simulink model "for_analysis"  (R2020a)
settings: Solver=VariableStepAuto  StartTime=0.0  StopTime=10.0  RelTol=1e-3
libraries: cstblocks x2
settings Model: Creator=Jason  LastModifiedBy=Jason

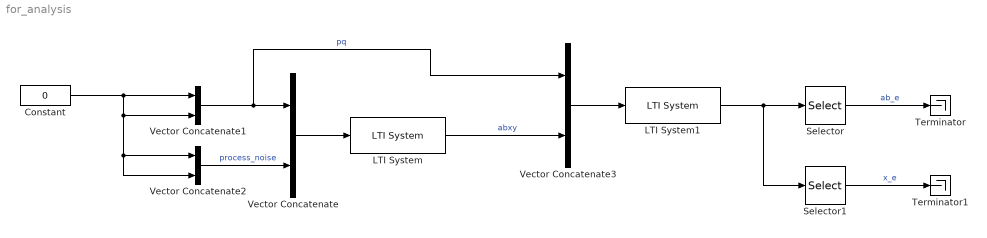
== system for_analysis ==
  Constant : Constant  Value=0
  LTI System : cstblocks/LTI System  sys=sys  IC=[]
  LTI System1 : cstblocks/LTI System  sys=kalmf  IC=[]
  Selector : Selector  InputPortWidth=4  IndexOptions=Index vector (dialog)  Indices=[1 2]  OutputSizes=1
  Selector1 : Selector  InputPortWidth=4  IndexOptions=Index vector (dialog)  Indices=[3 4]  OutputSizes=1
  Terminator : Terminator
  Terminator1 : Terminator
  Vector Concatenate{,1..3} (4 alike) : Concatenate
  wires:
  Vector Concatenate/1 -> LTI System/1
  Vector Concatenate1/1 -> Vector Concatenate3/1, Vector Concatenate/1  "pq"
  Vector Concatenate2/1 -> Vector Concatenate/2  "process_noise"
  Vector Concatenate3/1 -> LTI System1/1
  LTI System/1 -> Vector Concatenate3/2  "abxy"
  LTI System1/1 -> Selector1/1, Selector/1
  Selector/1 -> Terminator/1  "ab_e"
  Selector1/1 -> Terminator1/1  "x_e"
  Constant/1 -> Vector Concatenate2/2, Vector Concatenate2/1, Vector Concatenate1/2, Vector Concatenate1/1
